simulink model "pidwatertank"  (R2020a)
settings: Solver=FixedStepAuto  StartTime=0.0  StopTime=Tf  FixedStep=1  RelTol=1e-3  EnableMultiTasking=on
values from neighbouring files (symbols this model uses):
  F3_max = 1.01    [parameterpid.m]
  T2 = 25 + 273    (= 298)    [parameterpid.m]
  T4 = 37 + 273    (= 310)    [parameterpid.m]
settings Model: SimulationMode=accelerator  Creator=The MathWorks, Inc.  LastModifiedBy=ADMIN
settings DataIOCC: LimitDataPoints=on  SaveFormat=Array  ReturnWorkspaceOutputs=off  SignalLoggingName=logsOut
settings OptimizationCC: ExpressionDepthLimit=2147483647  InitFltsAndDblsToZero=on  LifeSpan=inf
settings DebuggingCC: SaveWithParameterizedLinksMsg=none  UnderspecifiedInitializationDetection=Classic  MergeDetectMultiDrivingBlocksExec=none  SignalResolutionControl=TryResolveAllWithWarning  MultiTaskDSMMsg=warning  FcnCallInpInsideContextMsg=warning  AllowSymbolicDim=off  StateNameClashWarn=warning  SFUnexpectedBacktrackingDiag=warning  SFNoUnconditionalDefaultTransitionDiag=warning  SFExecutionAtInitializationDiag=none  ArithmeticOperatorsInVariantConditions=warning
settings HardwareCC: ProdBitPerPointer=32  ProdBitPerSizeT=32  ProdBitPerPtrDiffT=32  ProdLargestAtomicFloat=None  ProdIntDivRoundTo=Undefined  ProdEndianess=Unspecified  ProdWordSize=32  ProdHWDeviceType=Specified
settings ModelReferenceCC: PropagateSignalLabelsOutOfModel=off
settings SFSimCC: SimUseLocalCustomCode=off  CustomCodeUndefinedFunction=UseInterfaceOnly
settings RTWCC: RTWUseLocalCustomCode=off
settings CodeAppCC: StateflowObjectComments=on
settings GRTTargetCC: TargetFcnLib=ansi_tfl_tmw.mat  TargetLangStandard=C89/C90 (ANSI)  CombineOutputUpdateFcns=off  GRTInterface=on
settings ConfigComp: CovMetricSettings=dw  CovHtmlReporting=on  CovSaveCumulativeToWorkspaceVar=on  CovSaveSingleToWorkspaceVar=on  CovExternalEMLEnable=off

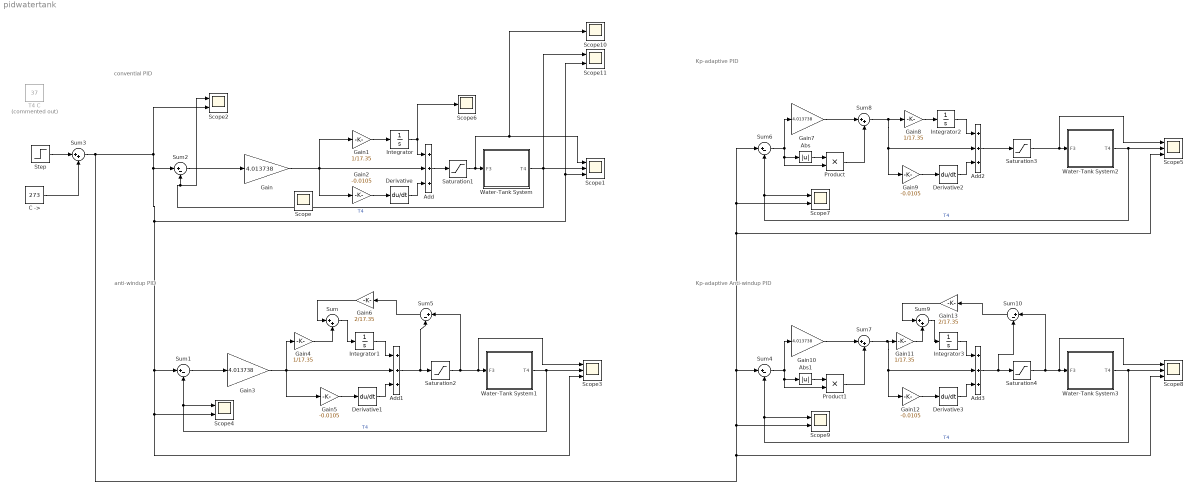
== system pidwatertank ==
  note: anti-windup PID
  note: convential PID
  note: Kp-adaptive PID
  note: Kp-adaptive Anti-windup PID
  Abs : Abs
  Abs1 : Abs
  Add{,1..3} (4 alike) : Sum  Inputs=+++
  "C ->  " : Constant  Value=273
  Derivative{,1..3} (4 alike) : Derivative
  Gain{,3,7,10} (4 alike) : Gain  Gain=4.013738
  Gain{1,4,8,11} (4 alike) : Gain  Gain=1/17.35
  Gain{2,5,9,12} (4 alike) : Gain  Gain=-0.0105
  Gain13 : Gain  Gain=2/17.35
  Gain6 : Gain  Gain=2/17.35
  Integrator{,1..3} (4 alike) : Integrator
  Product : Product
  Product1 : Product
  Saturation{1..4} (4 alike) : Saturate  UpperLimit=F3_max  LowerLimit=0
  Scope{1,3,5,8} (4 alike) : Scope  NumInputPorts=3
  Scope10 : Scope
  Scope{2,4,7,9,11} (5 alike) : Scope  NumInputPorts=2
  Scope6 : Scope
  Step : Step  Time=300  Before=37  After=40  SampleTime=0
  Sum{,3,7..9} (5 alike) : Sum  Inputs=|++
  Sum{1..2,4..6,10} (6 alike) : Sum  Inputs=|+-
  T4 C : Constant  Commented=on  Value=37
  Water-Tank System : Subsystem
  Water-Tank System1 : Subsystem
  Water-Tank System2 : Subsystem
  Water-Tank System3 : Subsystem
  Scope : Scope
  wires:
  Water-Tank System/1(T4) -> Scope11/1, Scope1/2, Scope2/1, Sum2/2  "T4"
  "C ->  "/1 -> Sum3/2
  Gain1/1 -> Integrator/1
  Gain2/1 -> Derivative/1
  Gain/1 -> Gain1/1, Add/2, Gain2/1
  Integrator/1 -> Add/1, Scope6/1
  Derivative/1 -> Add/3
  Sum2/1 -> Gain/1
  Add/1 -> Saturation1/1
  Add1/1 -> Saturation2/1, Sum5/2
  Sum1/1 -> Gain3/1
  Derivative1/1 -> Add1/3
  Integrator1/1 -> Add1/1
  Gain3/1 -> Gain4/1, Gain5/1, Add1/2
  Gain5/1 -> Derivative1/1
  Saturation2/1 -> Sum5/1, Water-Tank System1/1(F3), Scope3/1
  Water-Tank System1/1(T4) -> Sum1/2, Scope4/1, Scope3/2  "T4"
  Sum5/1 -> Gain6/1
  Sum/1 -> Integrator1/1
  Gain4/1 -> Sum/2
  Gain6/1 -> Sum/1
  Gain8/1 -> Integrator2/1
  Water-Tank System2/1(T4) -> Scope5/2, Sum6/2, Scope7/1  "T4"
  Saturation3/1 -> Scope5/1, Water-Tank System2/1(F3)
  Gain9/1 -> Derivative2/1
  Integrator2/1 -> Add2/1
  Derivative2/1 -> Add2/3
  Sum6/1 -> Gain7/1, Product/2, Abs/1
  Add2/1 -> Saturation3/1
  Gain7/1 -> Sum8/1
  Sum8/1 -> Add2/2, Gain9/1, Gain8/1
  Abs/1 -> Product/1
  Product/1 -> Sum8/2
  Product1/1 -> Sum7/2
  Abs1/1 -> Product1/1
  Sum7/1 -> Gain12/1, Add3/2, Gain11/1
  Gain10/1 -> Sum7/1
  Add3/1 -> Sum10/2, Saturation4/1
  Sum4/1 -> Abs1/1, Product1/2, Gain10/1
  Derivative3/1 -> Add3/3
  Integrator3/1 -> Add3/1
  Gain12/1 -> Derivative3/1
  Sum3/1 -> Sum6/1, Scope7/2, Scope5/3, Sum4/1, Scope9/2, Scope8/3, Scope11/2, Scope1/3, Scope3/3, Scope4/2, Sum1/1, Sum2/1, Scope2/2
  Saturation4/1 -> Sum10/1, Water-Tank System3/1(F3), Scope8/1
  Water-Tank System3/1(T4) -> Scope9/1, Sum4/2, Scope8/2  "T4"
  Gain11/1 -> Sum9/2
  Gain13/1 -> Sum9/1
  Sum9/1 -> Integrator3/1
  Sum10/1 -> Gain13/1
  Saturation1/1 -> Scope10/1, Scope1/1, Water-Tank System/1(F3)
  Step/1 -> Sum3/1

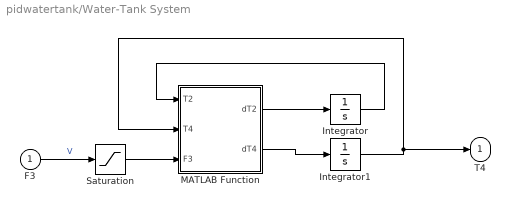
== system pidwatertank/Water-Tank System ==
  F3 : Inport
  Integrator : Integrator  InitialCondition=T2
  Integrator1 : Integrator  InitialCondition=T4
  MATLAB Function : MATLAB Function  TreatAsAtomicUnit=on
  Saturation : Saturate  UpperLimit=F3_max  LowerLimit=0
  T4 : Outport  VectorParamsAs1DForOutWhenUnconnected=off
  wires:
  MATLAB Function/1(dT2) -> Integrator/1
  MATLAB Function/2(dT4) -> Integrator1/1
  F3/1 -> Saturation/1  "V"
  Integrator/1 -> MATLAB Function/1(T2)
  Integrator1/1 -> MATLAB Function/2(T4), T4/1
  Saturation/1 -> MATLAB Function/3(F3)

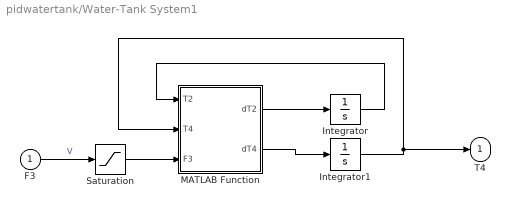
== system pidwatertank/Water-Tank System1 ==
  F3 : Inport
  Integrator : Integrator  InitialCondition=T2
  Integrator1 : Integrator  InitialCondition=T4
  MATLAB Function : MATLAB Function  TreatAsAtomicUnit=on
  Saturation : Saturate  UpperLimit=F3_max  LowerLimit=0
  T4 : Outport  VectorParamsAs1DForOutWhenUnconnected=off
  wires:
  Saturation/1 -> MATLAB Function/3(F3)
  Integrator1/1 -> T4/1, MATLAB Function/2(T4)
  Integrator/1 -> MATLAB Function/1(T2)
  F3/1 -> Saturation/1  "V"
  MATLAB Function/2(dT4) -> Integrator1/1
  MATLAB Function/1(dT2) -> Integrator/1

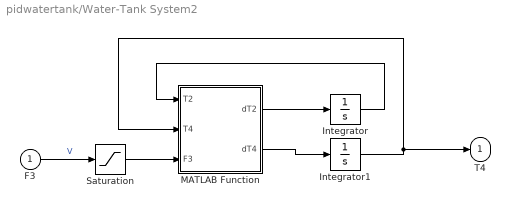
== system pidwatertank/Water-Tank System2 ==
  F3 : Inport
  Integrator : Integrator  InitialCondition=T2
  Integrator1 : Integrator  InitialCondition=T4
  MATLAB Function : MATLAB Function  TreatAsAtomicUnit=on
  Saturation : Saturate  UpperLimit=F3_max  LowerLimit=0
  T4 : Outport  VectorParamsAs1DForOutWhenUnconnected=off
  wires:
  MATLAB Function/1(dT2) -> Integrator/1
  MATLAB Function/2(dT4) -> Integrator1/1
  F3/1 -> Saturation/1  "V"
  Integrator/1 -> MATLAB Function/1(T2)
  Integrator1/1 -> MATLAB Function/2(T4), T4/1
  Saturation/1 -> MATLAB Function/3(F3)

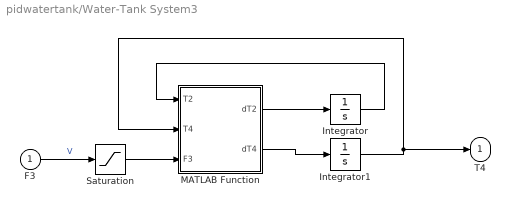
== system pidwatertank/Water-Tank System3 ==
  F3 : Inport
  Integrator : Integrator  InitialCondition=T2
  Integrator1 : Integrator  InitialCondition=T4
  MATLAB Function : MATLAB Function  TreatAsAtomicUnit=on
  Saturation : Saturate  UpperLimit=F3_max  LowerLimit=0
  T4 : Outport  VectorParamsAs1DForOutWhenUnconnected=off
  wires:
  Saturation/1 -> MATLAB Function/3(F3)
  Integrator1/1 -> T4/1, MATLAB Function/2(T4)
  Integrator/1 -> MATLAB Function/1(T2)
  F3/1 -> Saturation/1  "V"
  MATLAB Function/2(dT4) -> Integrator1/1
  MATLAB Function/1(dT2) -> Integrator/1

== matlab function pidwatertank/Water-Tank System1/MATLAB Function ==
  data: T2 input; dT2 output; T4 input; F3 input; dT4 output
function [dT2, dT4] = fcn(T2, T4, F3)
F1 = 0.5;           % m^3/s
T1 = 27+273;          % do Kevin
V1 = 100;               %  m^3
F3_max = 0.75;       % luu luong toi da cua F3 m^3/s
T3 = 50+273;          % do Kevin
V2 = 75;              % m^3   

dT2 = F1/V1 * (T1 - T2);
dT4 = F1/V2*(T2 - T4)+F3/V2*(T3-T4);

% [dT2 dT4] = [dT2_temp dT4_temp];

== matlab function pidwatertank/Water-Tank System/MATLAB Function ==
  data: T2 input; dT2 output; T4 input; F3 input; dT4 output
function [dT2, dT4] = fcn(T2, T4, F3)
F1 = 0.5;           % m^3/s
T1 = 27+273;          % do Kevin
V1 = 100;               %  m^3
F3_max = 1.01;       % luu luong toi da cua F3 m^3/s
T3 = 50+273;          % do Kevin
V2 = 75;              % m^3   

dT2 = F1/V1 * (T1 - T2);
dT4 = F1/V2*(T2 - T4)+F3/V2*(T3-T4);

% [dT2 dT4] = [dT2_temp dT4_temp];

== matlab function pidwatertank/Water-Tank System2/MATLAB Function ==
  data: T2 input; dT2 output; T4 input; F3 input; dT4 output
function [dT2, dT4] = fcn(T2, T4, F3)
F1 = 0.5;           % m^3/s
T1 = 27+273;          % do Kevin
V1 = 100;               %  m^3
F3_max = 0.75;       % luu luong toi da cua F3 m^3/s
T3 = 50+273;          % do Kevin
V2 = 75;              % m^3   

dT2 = F1/V1 * (T1 - T2);
dT4 = F1/V2*(T2 - T4)+F3/V2*(T3-T4);

% [dT2 dT4] = [dT2_temp dT4_temp];

== matlab function pidwatertank/Water-Tank System3/MATLAB Function ==
  data: T2 input; dT2 output; T4 input; F3 input; dT4 output
function [dT2, dT4] = fcn(T2, T4, F3)
F1 = 0.5;           % m^3/s
T1 = 27+273;          % do Kevin
V1 = 100;               %  m^3
F3_max = 0.75;       % luu luong toi da cua F3 m^3/s
T3 = 50+273;          % do Kevin
V2 = 75;              % m^3   

dT2 = F1/V1 * (T1 - T2);
dT4 = F1/V2*(T2 - T4)+F3/V2*(T3-T4);

% [dT2 dT4] = [dT2_temp dT4_temp];
